simulink model "problem3"  (R2017a)
settings: Solver=ode4  StartTime=0.0  StopTime=10  FixedStep=0.001  RelTol=1e-3
settings Model: Creator=donaghy1  LastModifiedBy=donaghy1

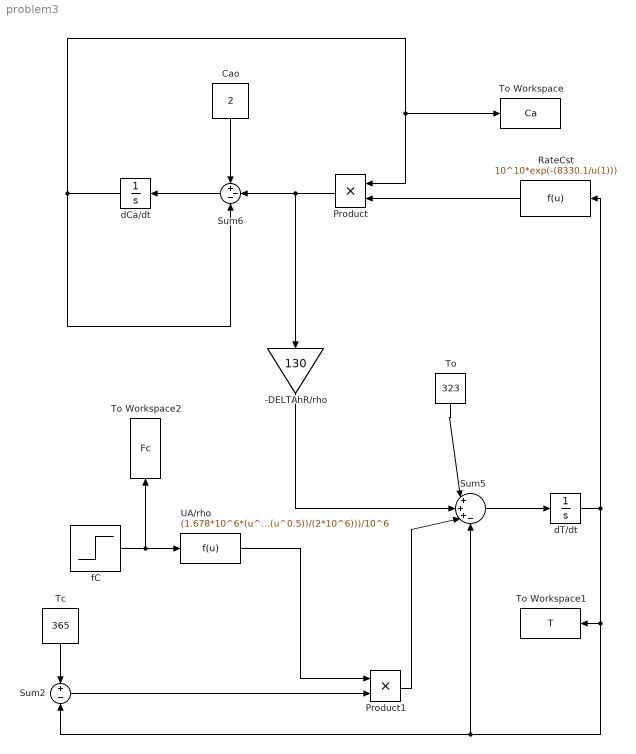
== system problem3 ==
  -DELTAhR/rho : Gain  Gain=130
  Cao : Constant  Value=2
  Product : Product
  Product1 : Product
  RateCst : Fcn  Expr=10^10*exp(-(8330.1/u(1)))
  Sum2 : Sum  Inputs=+-
  Sum5 : Sum  Inputs=|+++-
  Sum6 : Sum  Inputs=+--
  Tc : Constant  Value=365
  To : Constant  Value=323
  To Workspace : ToWorkspace  VariableName=Ca  SampleTime=-1
  To Workspace1 : ToWorkspace  VariableName=T  SampleTime=-1
  To Workspace2 : ToWorkspace  VariableName=Fc  SampleTime=-1
  UA/rho : Fcn  Expr=(1.678*10^6*(u^(1.5)))/(u+((1.678*10^6*(u^0.5))/(2*10^6)))/10^6
  dCa/dt : Integrator  InitialCondition=0.2646
  dT/dt : Integrator  InitialCondition=393.9521  AbsoluteTolerance=1000000
  fC : Step  Before=15  After=14  SampleTime=0
  wires:
  dCa/dt/1 -> Product/1, To Workspace/1, Sum6/3
  To/1 -> Sum5/1
  Tc/1 -> Sum2/1
  -DELTAhR/rho/1 -> Sum5/2
  Sum5/1 -> dT/dt/1
  Cao/1 -> Sum6/1
  Product/1 -> Sum6/2, -DELTAhR/rho/1
  Sum6/1 -> dCa/dt/1
  Product1/1 -> Sum5/3
  RateCst/1 -> Product/2
  Sum2/1 -> Product1/2
  UA/rho/1 -> Product1/1
  dT/dt/1 -> RateCst/1, Sum2/2, Sum5/4, To Workspace1/1
  fC/1 -> UA/rho/1, To Workspace2/1
